simulink library "Chassis_Alpha_sm_s3d"  (R2014a)
settings: Solver=ode45  StartTime=0.0  StopTime=10.0  RelTol=1e-3
undefined symbols (not defined in the file or in its folder): Chassis, open_system
libraries: Chassis_Alpha x2, Chassis_Alpha_sm x1, vrlib x1, simulink x1
Description:
  | Copyright 2013-2014 The MathWorks, Inc.
settings Model: Creator=mbrauer  LastModifiedBy=mbrauer

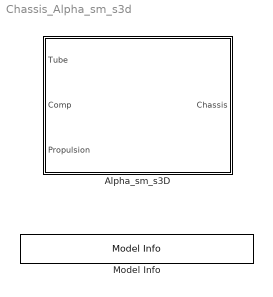
== system Chassis_Alpha_sm_s3d ==
  Alpha_sm_s3D : Subsystem  InitFcn=open_system([gcb,'/VR Sink'])
  Model Info : simulink/Model-Wide Utilities/Model Info  InitialBlockCM=None  BlockCM=none  Frame=on  DisplayStringWithTags=%<Description>  HorizontalTextAlignment=Center  LeftAlignmentValue=0.5  SourceBlockDiagram=Chassis_Alpha_sm_s3d  TagMaxNumber=20

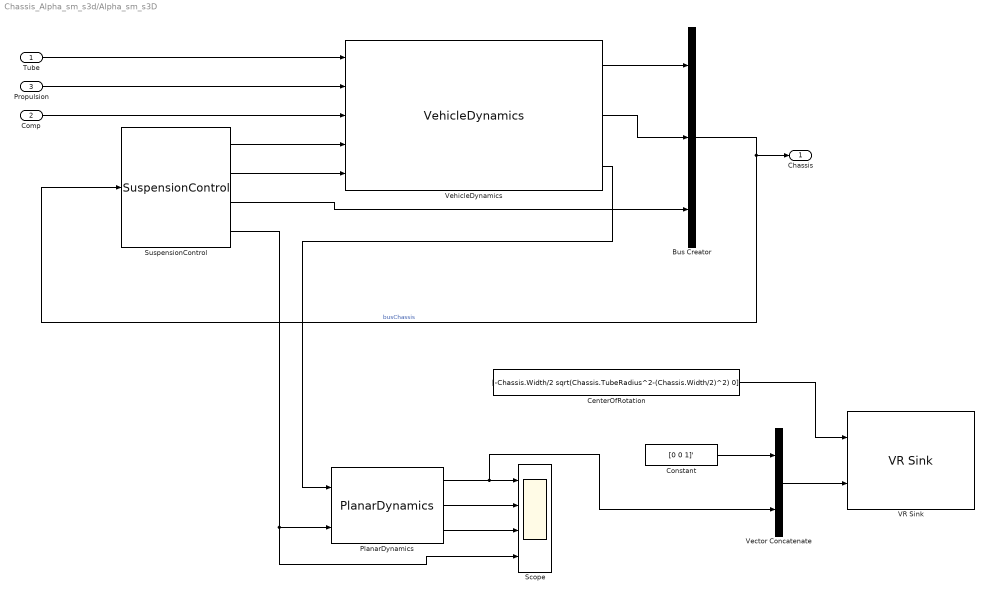
== system Chassis_Alpha_sm_s3d/Alpha_sm_s3D ==
  "Tube " : Inport
  Comp : Inport  Port=2
  Propulsion : Inport  Port=3
  Bus Creator : BusCreator  Inputs=3  NonVirtualBus=on
  CenterOfRotation : Constant  Value=[-Chassis.Width/2 sqrt(Chassis.TubeRadius^2-(Chassis.Width/2)^2) 0]'
  Constant : Constant  Value=[0 0 1]'
  PlanarDynamics : Chassis_Alpha_sm/PlanarDynamics  R=Chassis.TubeRadius  cH=Chassis.Height  cW=Chassis.Width  M=Chassis.Mass  D=5e3 % magic number
  Scope : Scope  NumInputPorts=4
      settings: YMin=-0.1~-12~-9.9~-5  YMax=0.55~2~-8.4~5  Decimation=10
  SuspensionControl : Chassis_Alpha/SuspensionControl
  VR Sink : vrlib/VR Sink  InstantiateOnLoad=on  SampleTime=0.1  ViewEnable=on  RemoteChange=off  RemoteView=off  FieldsWritten=HyperPod.center.3.1.1.double#HyperPod.rotation.4.1.1.double  WorldFileName=hyperLoopPod3D.wrl  AutoView=off  VideoDimensions=[]  AllowVariableSize=off
  Vector Concatenate : Concatenate
  VehicleDynamics : Chassis_Alpha/VehicleDynamics
  Chassis : Outport
  wires:
  VehicleDynamics/3 -> PlanarDynamics/1
  SuspensionControl/4 -> PlanarDynamics/2, Scope/4
  PlanarDynamics/3 -> Scope/3
  PlanarDynamics/2 -> Scope/2
  Vector Concatenate/1 -> VR Sink/2
  CenterOfRotation/1 -> VR Sink/1
  Constant/1 -> Vector Concatenate/1
  PlanarDynamics/1 -> Scope/1, Vector Concatenate/2
  Bus Creator/1 -> SuspensionControl/1, Chassis/1  "busChassis"
  Comp/1 -> VehicleDynamics/3
  "Tube "/1 -> VehicleDynamics/1
  VehicleDynamics/1 -> Bus Creator/1
  VehicleDynamics/2 -> Bus Creator/2
  Propulsion/1 -> VehicleDynamics/2
  SuspensionControl/1 -> VehicleDynamics/4
  SuspensionControl/2 -> VehicleDynamics/5
  SuspensionControl/3 -> Bus Creator/3
